simulink model "Systems_simulation"  (R2020a)
settings: Solver=VariableStepAuto  StartTime=0.0  StopTime=15000  MaxStep=0.1  RelTol=1e-3
undefined symbols (not defined in the file): a, b, Qin_1, Qin_2
libraries: cstblocks x18
settings Model: Creator=beto1  LastModifiedBy=beto1

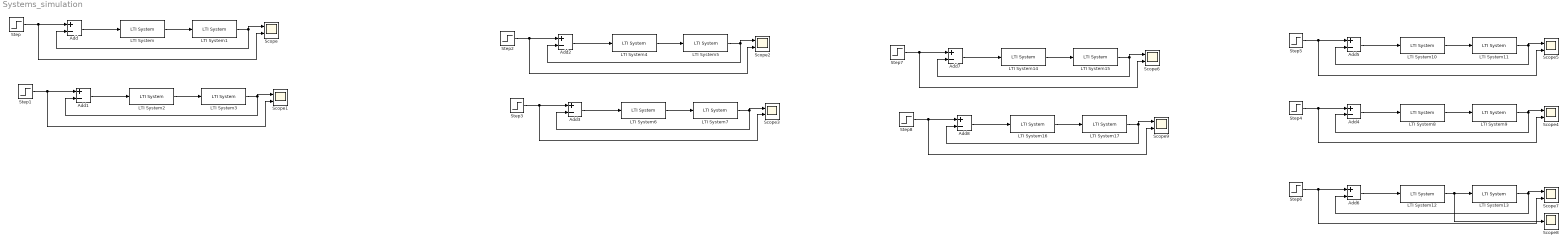
== system Systems_simulation ==
  Add{,1..8} (9 alike) : Sum  Inputs=+-
  LTI System : cstblocks/LTI System  sys=C1  IC=[]
  LTI System1 : cstblocks/LTI System  sys=G1  IC=[]
  LTI System10 : cstblocks/LTI System  sys=C5_H1  IC=[]
  LTI System11 : cstblocks/LTI System  sys=H1  IC=[]
  LTI System12 : cstblocks/LTI System  sys=C5_C  IC=[]
  LTI System13 : cstblocks/LTI System  sys=H2  IC=[]
  LTI System14 : cstblocks/LTI System  sys=C3  IC=[]
  LTI System15 : cstblocks/LTI System  sys=G3  IC=[]
  LTI System16 : cstblocks/LTI System  sys=C3_C  IC=[]
  LTI System17 : cstblocks/LTI System  sys=G3  IC=[]
  LTI System2 : cstblocks/LTI System  sys=C1_C  IC=[]
  LTI System3 : cstblocks/LTI System  sys=G1  IC=[]
  LTI System4 : cstblocks/LTI System  sys=C2  IC=[]
  LTI System5 : cstblocks/LTI System  sys=G2  IC=[]
  LTI System6 : cstblocks/LTI System  sys=C2_C  IC=[]
  LTI System7 : cstblocks/LTI System  sys=G2  IC=[]
  LTI System8 : cstblocks/LTI System  sys=C5_H2  IC=[]
  LTI System9 : cstblocks/LTI System  sys=H2  IC=[]
  Scope{,1..7,9} (9 alike) : Scope  NumInputPorts=2
  Scope8 : Scope
  Step : Step  Time=0  After=a  SampleTime=0
  Step1 : Step  Time=0  After=b  SampleTime=0
  Step2 : Step  Time=0  After=a  SampleTime=0
  Step3 : Step  Time=0  After=b  SampleTime=0
  Step4 : Step  Time=0  After=Qin_2  SampleTime=0
  Step5 : Step  Time=0  After=Qin_1  SampleTime=0
  Step6 : Step  Time=0  After=Qin_2  SampleTime=0
  Step7 : Step  Time=0  After=a  SampleTime=0
  Step8 : Step  Time=0  After=b  SampleTime=0
  wires:
  Step/1 -> Scope/2, Add/1
  LTI System/1 -> LTI System1/1
  Add/1 -> LTI System/1
  LTI System1/1 -> Add/2, Scope/1
  Add1/1 -> LTI System2/1
  Step1/1 -> Scope1/2, Add1/1
  LTI System2/1 -> LTI System3/1
  LTI System3/1 -> Add1/2, Scope1/1
  LTI System4/1 -> LTI System5/1
  Add2/1 -> LTI System4/1
  Step2/1 -> Scope2/2, Add2/1
  LTI System5/1 -> Add2/2, Scope2/1
  Step3/1 -> Scope3/2, Add3/1
  Add3/1 -> LTI System6/1
  LTI System7/1 -> Add3/2, Scope3/1
  LTI System6/1 -> LTI System7/1
  Step4/1 -> Scope4/2, Add4/1
  LTI System9/1 -> Add4/2, Scope4/1
  Add4/1 -> LTI System8/1
  LTI System8/1 -> LTI System9/1
  Step5/1 -> Scope5/2, Add5/1
  LTI System11/1 -> Add5/2, Scope5/1
  Add5/1 -> LTI System10/1
  LTI System10/1 -> LTI System11/1
  LTI System12/1 -> Scope8/1, LTI System13/1
  Step6/1 -> Scope7/2, Add6/1
  Add6/1 -> LTI System12/1
  LTI System13/1 -> Add6/2, Scope7/1
  Add8/1 -> LTI System16/1
  LTI System16/1 -> LTI System17/1
  LTI System17/1 -> Add8/2, Scope9/1
  Step8/1 -> Scope9/2, Add8/1
  LTI System14/1 -> LTI System15/1
  LTI System15/1 -> Add7/2, Scope6/1
  Add7/1 -> LTI System14/1
  Step7/1 -> Scope6/2, Add7/1
